simulink model "gaussian_filter_v2"  (R2020b)
settings: Solver=VariableStepAuto  StartTime=0.0  StopTime=2  RelTol=1e-3
values from neighbouring files (symbols this model uses):
  COLS = 752    [setup.m]
libraries: hdlsllib x3, visionhdlio x2, visionsources x1
settings Model: FPTShortcutValueString='{{},{''BaselineRun_2'',1,1,1,''BaselineRun_2'','''',{},''M'','''',''''},{''BaselineRun_3'',1,1,1,''BaselineRun_3'','''',{},''M'','''',''''},{''BaselineRun_4'',1,1,1,''BaselineRun_4'','''',{},''M'','''',''''}}'  Creator=Ethan  LastModifiedBy=Ethan
settings DebuggingCC: SignalRangeChecking=warning

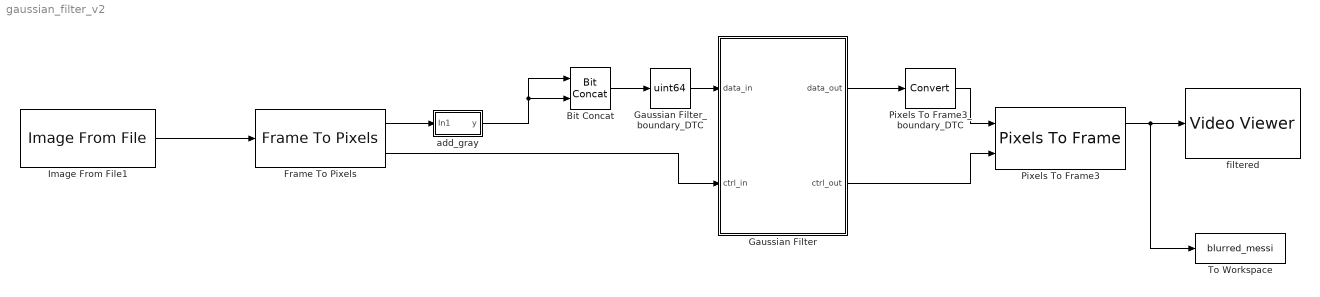
== system gaussian_filter_v2 ==
  Bit Concat : hdlsllib/Logic and Bit Operations/Bit Concat  numInputs=2
  Frame To Pixels : visionhdlio/Frame To Pixels  NumComponents=3  NumPixels=1  VideoFormat=Custom  ActivePixelsPerLine=752  ActiveVideoLines=480  TotalPixelsPerLine=752  TotalVideoLines=480  StartingActiveLine=1  FrontPorch=0  SampleTime=0
      settings: SourceProductName=Vision HDL Toolbox
  Gaussian Filter : Subsystem
  Gaussian Filter_boundary_DTC : DataTypeConversion  OutDataTypeStr=uint64  SaturateOnIntegerOverflow=on  RndMeth=Zero
  Image From File1 : visionsources/Image From File  Tag=vipblks_nd  FileName=messi.jpg  Ts=1  imagePorts=One multidimensional signal  OutPortLabels=R|G|B  ImageDataType=uint8  sdImageDataType=uint(8)  Signed=on  WordLength=16  FractionLengthMode=User-defined  FractionLength=15
  Pixels To Frame3 : visionhdlio/Pixels To Frame  NumComponents=1  NumPixels=1  VideoFormat=Custom  ActivePixelsPerLine=752  ActiveVideoLines=480  TotalPixelsPerLine=752  TotalVideoLines=480
      settings: SourceProductBaseCode=VT
  Pixels To Frame3_boundary_DTC : DataTypeConversion  SaturateOnIntegerOverflow=on  RndMeth=Zero
  To Workspace : ToWorkspace  VariableName=blurred_messi  SaveFormat=Timeseries  SampleTime=-1
  add_gray : Subsystem
  filtered : VideoViewer  FigPos=[441 938 1280 623]
  wires:
  Pixels To Frame3/1 -> To Workspace/1, filtered/1
  Gaussian Filter/2(ctrl_out) -> Pixels To Frame3/2
  Gaussian Filter/1(data_out) -> Pixels To Frame3_boundary_DTC/1
  Pixels To Frame3_boundary_DTC/1 -> Pixels To Frame3/1
  Bit Concat/1 -> Gaussian Filter_boundary_DTC/1
  Gaussian Filter_boundary_DTC/1 -> Gaussian Filter/1(data_in)
  Frame To Pixels/2 -> Gaussian Filter/2(ctrl_in)
  Image From File1/1 -> Frame To Pixels/1
  add_gray/1(y) -> Bit Concat/1, Bit Concat/2
  Frame To Pixels/1 -> add_gray/1(In1)

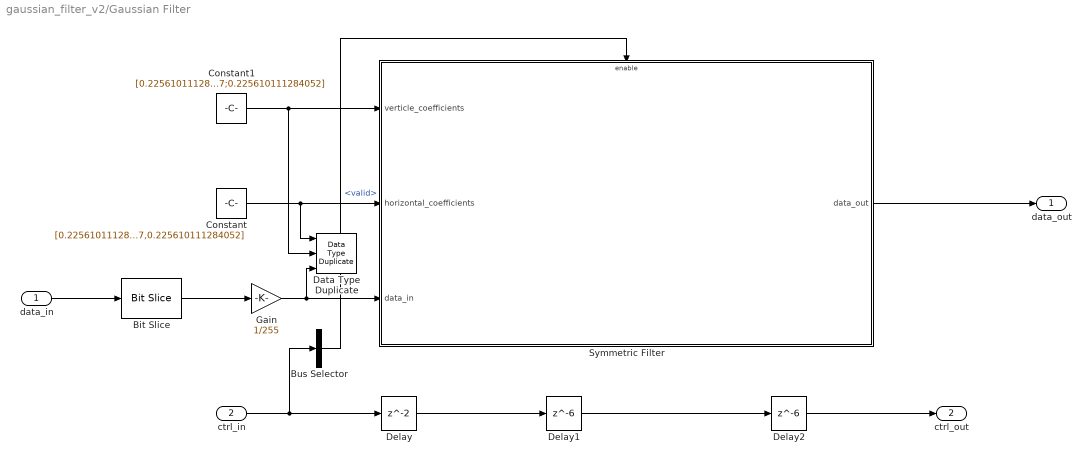
== system gaussian_filter_v2/Gaussian Filter ==
  data_in : Inport
  ctrl_in : Inport  Port=2
  Bit Slice : hdlsllib/Logic and Bit Operations/Bit Slice  lidx=31  ridx=24
      settings: SourceProductBaseCode=SL
  Bus Selector : BusSelector  OutputSignals=valid
  Constant : Constant  Value=[0.225610111284052,0.548779777431897,0.225610111284052]  OutDataTypeStr=Inherit: Inherit via back propagation  SampleTime=-1
  Constant1 : Constant  Value=[0.225610111284051;0.548779777431897;0.225610111284052]  OutDataTypeStr=Inherit: Inherit via back propagation  SampleTime=-1
  Data Type Duplicate : DataTypeDuplicate  NumInputPorts=3
  Delay : Delay
  Delay1 : Delay  DelayLength=6
  Delay2 : Delay  DelayLength=6
  Gain : Gain  Gain=1/255  OutDataTypeStr=cap_1
  Symmetric Filter : Subsystem
  data_out : Outport
  ctrl_out : Outport  Port=2
  wires:
  ctrl_in/1 -> Bus Selector/1, Delay/1
  Delay/1 -> Delay1/1
  Delay1/1 -> Delay2/1
  Delay2/1 -> ctrl_out/1
  data_in/1 -> Bit Slice/1
  Bus Selector/1 -> Symmetric Filter/Enable  "<valid>"
  Constant/1 -> Data Type Duplicate/1, Symmetric Filter/2(horizontal_coefficients)
  Constant1/1 -> Data Type Duplicate/2, Symmetric Filter/1(verticle_coefficients)
  Bit Slice/1 -> Gain/1
  Gain/1 -> Data Type Duplicate/3, Symmetric Filter/3(data_in)
  Symmetric Filter/1(data_out) -> data_out/1

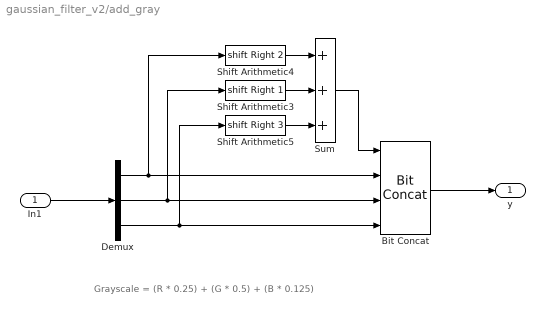
== system gaussian_filter_v2/add_gray ==
  note: Grayscale = (R * 0.25) + (G * 0.5) + (B * 0.125)
  In1 : Inport
  Bit Concat : hdlsllib/Logic and Bit Operations/Bit Concat  numInputs=4
  Demux : Demux  Outputs=3
  Shift Arithmetic3 : ArithShift  BitShiftNumber=1  BitShiftDirection=Right
  Shift Arithmetic4 : ArithShift  BitShiftNumber=2  BitShiftDirection=Right
  Shift Arithmetic5 : ArithShift  BitShiftNumber=3  BitShiftDirection=Right
  Sum : Sum  Inputs=+++  OutDataTypeStr=uint8
  y : Outport
  wires:
  Bit Concat/1 -> y/1
  In1/1 -> Demux/1
  Demux/2 -> Shift Arithmetic3/1, Bit Concat/3
  Demux/1 -> Shift Arithmetic4/1, Bit Concat/2
  Demux/3 -> Shift Arithmetic5/1, Bit Concat/4
  Sum/1 -> Bit Concat/1
  Shift Arithmetic4/1 -> Sum/1
  Shift Arithmetic3/1 -> Sum/2
  Shift Arithmetic5/1 -> Sum/3

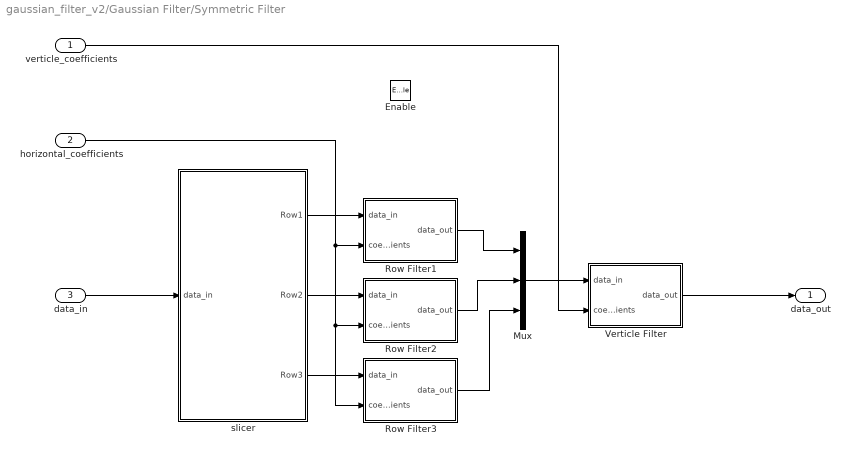
== system gaussian_filter_v2/Gaussian Filter/Symmetric Filter ==
  verticle_coefficients : Inport
  horizontal_coefficients : Inport  Port=2
  data_in : Inport  Port=3
  Enable : EnablePort
  Mux : Mux  Inputs=3
  Row Filter1 : Subsystem
  Row Filter2 : Subsystem
  Row Filter3 : Subsystem
  Verticle Filter : Subsystem
  slicer : Subsystem
  data_out : Outport
  wires:
  Row Filter2/1(data_out) -> Mux/2
  Row Filter3/1(data_out) -> Mux/3
  Row Filter1/1(data_out) -> Mux/1
  slicer/1(Row1) -> Row Filter1/1(data_in)
  data_in/1 -> slicer/1(data_in)
  horizontal_coefficients/1 -> Row Filter3/2(coefficients), Row Filter2/2(coefficients), Row Filter1/2(coefficients)
  slicer/2(Row2) -> Row Filter2/1(data_in)
  slicer/3(Row3) -> Row Filter3/1(data_in)
  Mux/1 -> Verticle Filter/1(data_in)
  Verticle Filter/1(data_out) -> data_out/1
  verticle_coefficients/1 -> Verticle Filter/2(coefficients)

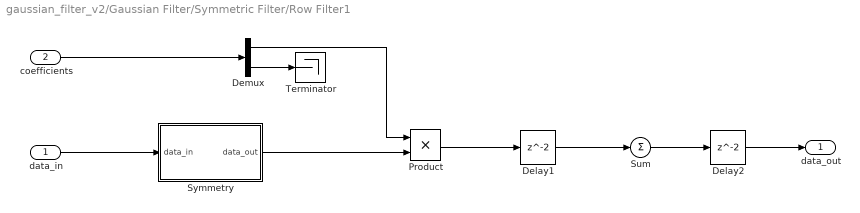
== system gaussian_filter_v2/Gaussian Filter/Symmetric Filter/Row Filter1 ==
  data_in : Inport
  coefficients : Inport  Port=2
  Delay1 : Delay
  Delay2 : Delay
  Demux : Demux  Outputs=[2, 1]
  Product : Product  OutDataTypeStr=cap_1
  Sum : Sum  Inputs=1  AccumDataTypeStr=cap_1  OutDataTypeStr=cap_1
  Symmetry : Subsystem
  Terminator : Terminator
  data_out : Outport
  wires:
  Product/1 -> Delay1/1
  Symmetry/1(data_out) -> Product/2
  Delay1/1 -> Sum/1
  Delay2/1 -> data_out/1
  Sum/1 -> Delay2/1
  data_in/1 -> Symmetry/1(data_in)
  coefficients/1 -> Demux/1
  Demux/1 -> Product/1
  Demux/2 -> Terminator/1

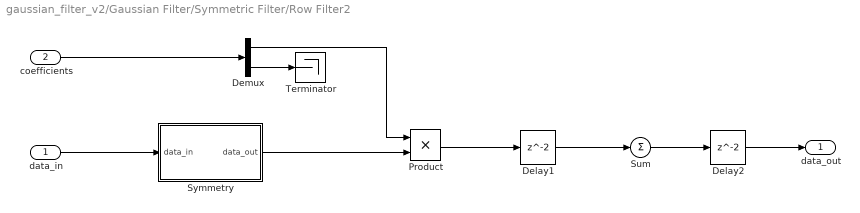
== system gaussian_filter_v2/Gaussian Filter/Symmetric Filter/Row Filter2 ==
  data_in : Inport
  coefficients : Inport  Port=2
  Delay1 : Delay
  Delay2 : Delay
  Demux : Demux  Outputs=[2, 1]
  Product : Product  OutDataTypeStr=cap_1
  Sum : Sum  Inputs=1  AccumDataTypeStr=cap_1  OutDataTypeStr=cap_1
  Symmetry : Subsystem
  Terminator : Terminator
  data_out : Outport
  wires:
  Product/1 -> Delay1/1
  Symmetry/1(data_out) -> Product/2
  Delay1/1 -> Sum/1
  Delay2/1 -> data_out/1
  Sum/1 -> Delay2/1
  data_in/1 -> Symmetry/1(data_in)
  coefficients/1 -> Demux/1
  Demux/1 -> Product/1
  Demux/2 -> Terminator/1

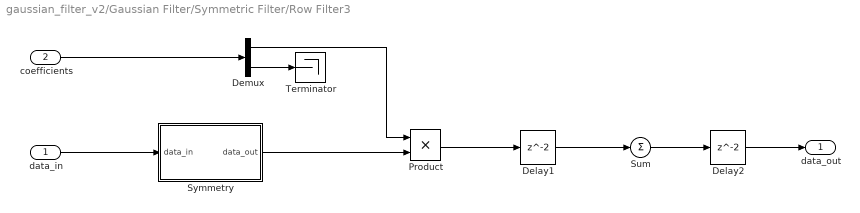
== system gaussian_filter_v2/Gaussian Filter/Symmetric Filter/Row Filter3 ==
  data_in : Inport
  coefficients : Inport  Port=2
  Delay1 : Delay
  Delay2 : Delay
  Demux : Demux  Outputs=[2, 1]
  Product : Product  OutDataTypeStr=cap_1
  Sum : Sum  Inputs=1  AccumDataTypeStr=cap_1  OutDataTypeStr=cap_1
  Symmetry : Subsystem
  Terminator : Terminator
  data_out : Outport
  wires:
  Product/1 -> Delay1/1
  Symmetry/1(data_out) -> Product/2
  Delay1/1 -> Sum/1
  Delay2/1 -> data_out/1
  Sum/1 -> Delay2/1
  data_in/1 -> Symmetry/1(data_in)
  coefficients/1 -> Demux/1
  Demux/1 -> Product/1
  Demux/2 -> Terminator/1

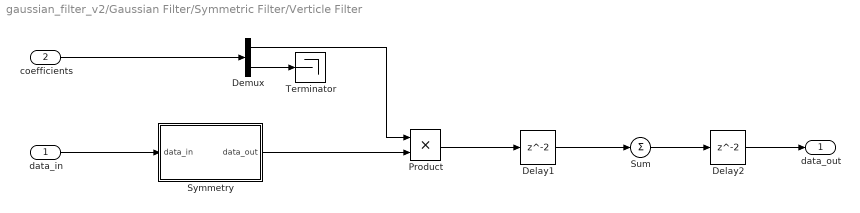
== system gaussian_filter_v2/Gaussian Filter/Symmetric Filter/Verticle Filter ==
  data_in : Inport
  coefficients : Inport  Port=2
  Delay1 : Delay
  Delay2 : Delay
  Demux : Demux  Outputs=[2, 1]
  Product : Product  OutDataTypeStr=cap_1
  Sum : Sum  Inputs=1  AccumDataTypeStr=cap_1  OutDataTypeStr=cap_1
  Symmetry : Subsystem
  Terminator : Terminator
  data_out : Outport
  wires:
  Product/1 -> Delay1/1
  Symmetry/1(data_out) -> Product/2
  Delay1/1 -> Sum/1
  Delay2/1 -> data_out/1
  Sum/1 -> Delay2/1
  data_in/1 -> Symmetry/1(data_in)
  coefficients/1 -> Demux/1
  Demux/1 -> Product/1
  Demux/2 -> Terminator/1

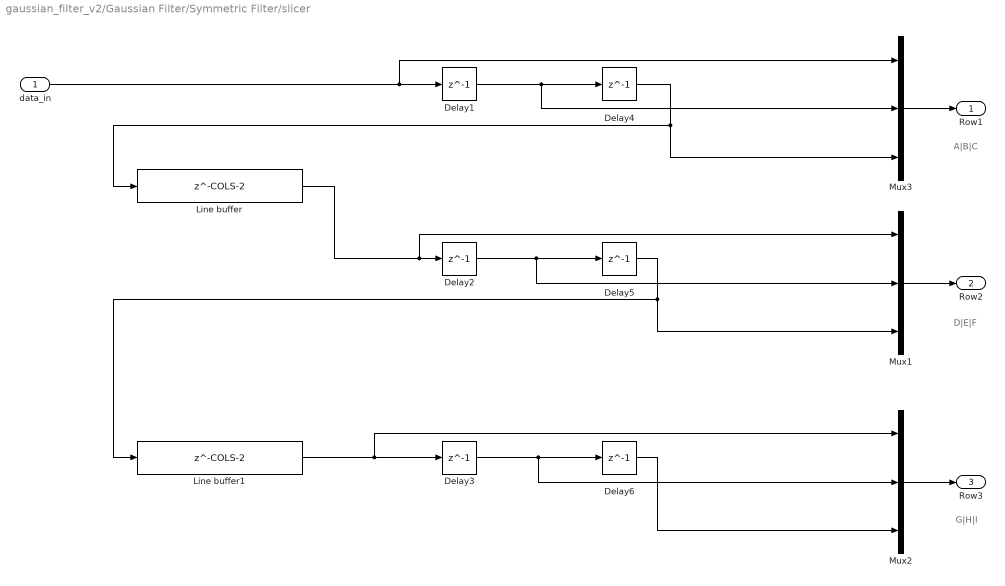
== system gaussian_filter_v2/Gaussian Filter/Symmetric Filter/slicer ==
  note: A|B|C
  note: D|E|F
  note: G|H|I
  data_in : Inport
  Delay{1..6} (6 alike) : Delay  DelayLength=1  InitialCondition=0
  Line buffer : Delay  DelayLength=COLS-2  InitialCondition=0
  Line buffer1 : Delay  DelayLength=COLS-2  InitialCondition=0
  Mux1 : Mux  Inputs=3
  Mux2 : Mux  Inputs=3
  Mux3 : Mux  Inputs=3
  Row1 : Outport  VectorParamsAs1DForOutWhenUnconnected=off
  Row2 : Outport  Port=2  VectorParamsAs1DForOutWhenUnconnected=off
  Row3 : Outport  Port=3  VectorParamsAs1DForOutWhenUnconnected=off
  wires:
  Delay4/1 -> Mux3/3, Line buffer/1
  data_in/1 -> Mux3/1, Delay1/1
  Delay1/1 -> Mux3/2, Delay4/1
  Delay3/1 -> Mux2/2, Delay6/1
  Delay5/1 -> Mux1/3, Line buffer1/1
  Delay6/1 -> Mux2/3
  Line buffer/1 -> Mux1/1, Delay2/1
  Line buffer1/1 -> Mux2/1, Delay3/1
  Delay2/1 -> Mux1/2, Delay5/1
  Mux1/1 -> Row2/1
  Mux2/1 -> Row3/1
  Mux3/1 -> Row1/1

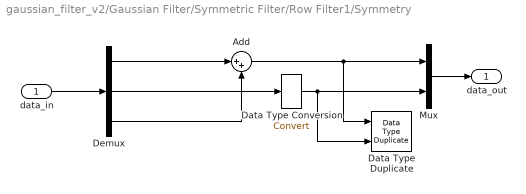
== system gaussian_filter_v2/Gaussian Filter/Symmetric Filter/Row Filter1/Symmetry ==
  data_in : Inport
  Add : Sum  Inputs=|++  AccumDataTypeStr=cap_2  OutDataTypeStr=cap_2  RndMeth=Nearest
  Data Type Duplicate : DataTypeDuplicate
  Data Type Conversion : DataTypeConversion
  Demux : Demux  Outputs=3
  Mux : Mux  Inputs=2
  data_out : Outport
  wires:
  Add/1 -> Data Type Duplicate/1, Mux/1
  data_in/1 -> Demux/1
  Demux/3 -> Add/2
  Demux/1 -> Add/1
  Mux/1 -> data_out/1
  Demux/2 -> Data Type Conversion/1
  Data Type Conversion/1 -> Data Type Duplicate/2, Mux/2

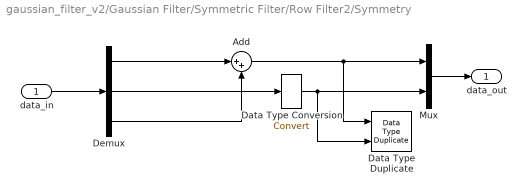
== system gaussian_filter_v2/Gaussian Filter/Symmetric Filter/Row Filter2/Symmetry ==
  data_in : Inport
  Add : Sum  Inputs=|++  AccumDataTypeStr=cap_2  OutDataTypeStr=cap_2  RndMeth=Nearest
  Data Type Duplicate : DataTypeDuplicate
  Data Type Conversion : DataTypeConversion
  Demux : Demux  Outputs=3
  Mux : Mux  Inputs=2
  data_out : Outport
  wires:
  Add/1 -> Data Type Duplicate/1, Mux/1
  data_in/1 -> Demux/1
  Demux/3 -> Add/2
  Demux/1 -> Add/1
  Mux/1 -> data_out/1
  Demux/2 -> Data Type Conversion/1
  Data Type Conversion/1 -> Data Type Duplicate/2, Mux/2

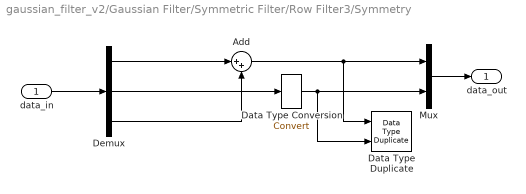
== system gaussian_filter_v2/Gaussian Filter/Symmetric Filter/Row Filter3/Symmetry ==
  data_in : Inport
  Add : Sum  Inputs=|++  AccumDataTypeStr=cap_2  OutDataTypeStr=cap_2  RndMeth=Nearest
  Data Type Duplicate : DataTypeDuplicate
  Data Type Conversion : DataTypeConversion
  Demux : Demux  Outputs=3
  Mux : Mux  Inputs=2
  data_out : Outport
  wires:
  Add/1 -> Data Type Duplicate/1, Mux/1
  data_in/1 -> Demux/1
  Demux/3 -> Add/2
  Demux/1 -> Add/1
  Mux/1 -> data_out/1
  Demux/2 -> Data Type Conversion/1
  Data Type Conversion/1 -> Data Type Duplicate/2, Mux/2

== system gaussian_filter_v2/Gaussian Filter/Symmetric Filter/Verticle Filter/Symmetry ==
  data_in : Inport
  Add : Sum  Inputs=|++  AccumDataTypeStr=cap_2  OutDataTypeStr=cap_2  RndMeth=Nearest
  Data Type Duplicate : DataTypeDuplicate
  Data Type Conversion : DataTypeConversion
  Demux : Demux  Outputs=3
  Mux : Mux  Inputs=2
  data_out : Outport
  wires:
  Add/1 -> Data Type Duplicate/1, Mux/1
  data_in/1 -> Demux/1
  Demux/3 -> Add/2
  Demux/1 -> Add/1
  Mux/1 -> data_out/1
  Demux/2 -> Data Type Conversion/1
  Data Type Conversion/1 -> Data Type Duplicate/2, Mux/2
